simulink model "i2c_logger"  (R2021b)
settings: Solver=FixedStepAuto  StartTime=0.0  StopTime=10.0  RelTol=1e-3  EnableMultiTasking=on
libraries: mbedblockslib x8, simulink x2, realtime_examples_misc x1
settings Model: ExtModeTrigDuration=10  Creator=Robert Viramontes  LastModifiedBy=Robert Viramontes
settings OptimizationCC: EnhancedBackFolding=on  PassReuseOutputArgsAs=Individual arguments  ZeroExternalMemoryAtStartup=off  ZeroInternalMemoryAtStartup=off  MaxStackSize=64  OptimizeBlockOrder=speed  DifferentSizesBufferReuse=on  OptimizationCustomize=off  EfficientTunableParamExpr=on
settings DebuggingCC: ParameterTunabilityLossMsg=error
settings HardwareCC: ProdBitPerPointer=32  ProdBitPerSizeT=32  ProdBitPerPtrDiffT=32  ProdLargestAtomicInteger=Long  ProdLargestAtomicFloat=Double  ProdWordSize=32  ProdHWDeviceType=ARM Compatible->ARM Cortex
settings SFSimCC: MATLABDynamicMemAlloc=off
settings RTWCC: Description=Embedded Coder  SystemTargetFile=ert.tlc  HardwareBoard=STM32 Nucleo F411RE  TemplateMakefile=ert_default_tmf  Toolchain=GNU Tools for ARM Embedded Processors
settings CodeAppCC: ForceParamTrailComments=on  IgnoreCustomStorageClasses=off  OperatorAnnotations=on  SimulinkDataObjDesc=on  SFDataObjDesc=on  InsertBlockDesc=on
settings ERTTargetCC: ExtModeTransport=3  ExtModeStaticAlloc=on  ExtModeStaticAllocSize=2000  ExtModeMexFile=ext_xcp  ExtModeIntrfLevel=Level2 - Open

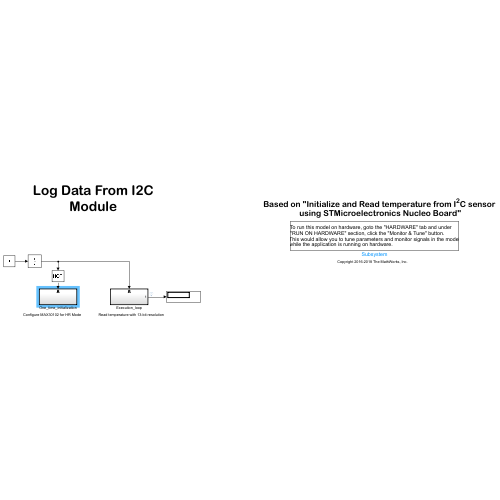
[thumbnail: Simulink's stored preview of the top-level diagram]
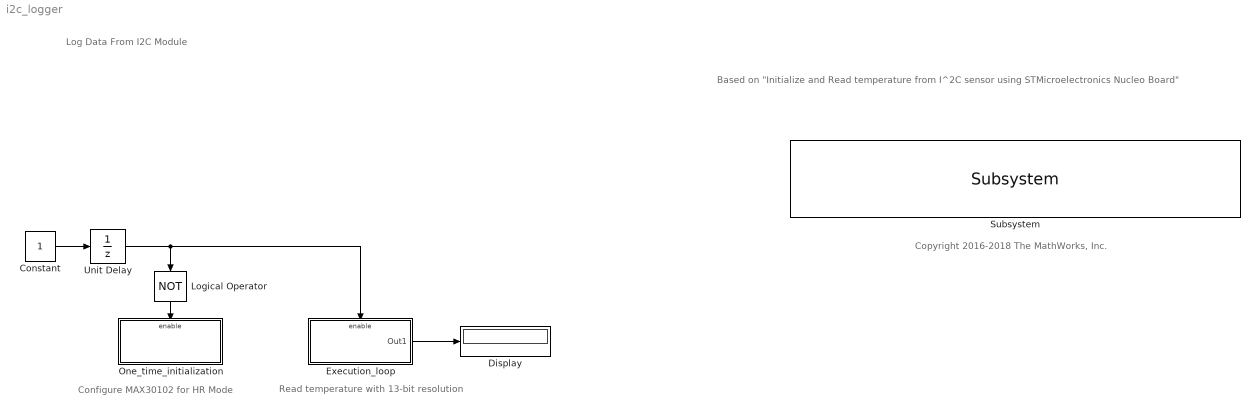
== system i2c_logger ==
  note: Log Data From I2C Module
  note: Read temperature with 13-bit resolution
  note: Configure MAX30102 for HR Mode
  note: Copyright 2016-2018 The MathWorks, Inc.
  note: Based on "Initialize and Read temperature from I^2C sensor
      |  using STMicroelectronics Nucleo Board"
  Constant : Constant  OutDataTypeStr=boolean  SampleTime=0.1
  Display : Display
      settings: Format=hex (Stored Integer)
  Execution_loop : Subsystem  TreatAsAtomicUnit=on
  Logical Operator : Logic  Operator=NOT  AllPortsSameDT=off  OutDataTypeStr=boolean
  One_time_initialization : Subsystem  TreatAsAtomicUnit=on
  Subsystem : realtime_examples_misc/Subsystem  SystemSampleTime=-1  VariantActivationTime=update diagram  Latency=0  AutoFrameSizeCalculation=off
      settings: SourceProductBaseCode=SL
  Unit Delay : UnitDelay  SampleTime=-1  HasFrameUpgradeWarning=on
  wires:
  Logical Operator/1 -> One_time_initialization/Enable
  Execution_loop/1(Out1) -> Display/1
  Constant/1 -> Unit Delay/1
  Unit Delay/1 -> Execution_loop/Enable, Logical Operator/1

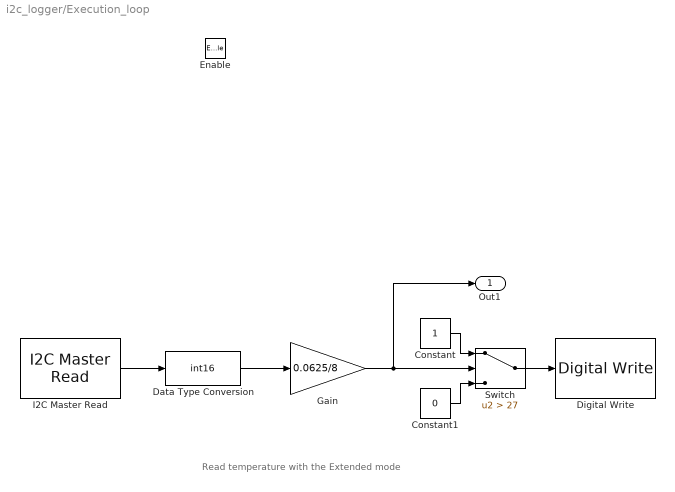
== system i2c_logger/Execution_loop ==
  note: Read temperature with the Extended mode
  Enable : EnablePort
  Constant : Constant  OutDataTypeStr=uint8
  Constant1 : Constant  Value=0  OutDataTypeStr=uint8
  Data Type Conversion : DataTypeConversion  OutDataTypeStr=int16  ConvertRealWorld=Stored Integer (SI)
  Digital Write : mbedblockslib/Digital Write  Pin=13  Direction=output
      settings: SourceProductBaseCode=MICROBIT,NUCLEO,STMICRODIS
  Gain : Gain  Gain=0.0625/8  OutDataTypeStr=single
  I2C Master Read : mbedblockslib/I2C Master Read  I2CModule=0  Mode=Master  SlaveAddress=hex2dec('48')  SlaveByteOrder=BigEndian  Direction=Receiver  RegisterAddressMode=on  RegisterAddress=uint8(0)  SlaveDataType=uint16  DataLength=1  NoAck=off  RepeatedStart=off  OutputStatus=off  SampleTime=0.1
      settings: SourceProductBaseCode=MICROBIT,NUCLEO,STMICRODIS
  Switch : Switch  Criteria=u2 > Threshold  Threshold=27
  Out1 : Outport  InitialOutput=0  VectorParamsAs1DForOutWhenUnconnected=off
  wires:
  I2C Master Read/1 -> Data Type Conversion/1
  Data Type Conversion/1 -> Gain/1
  Gain/1 -> Out1/1, Switch/2
  Constant/1 -> Switch/1
  Constant1/1 -> Switch/3
  Switch/1 -> Digital Write/1

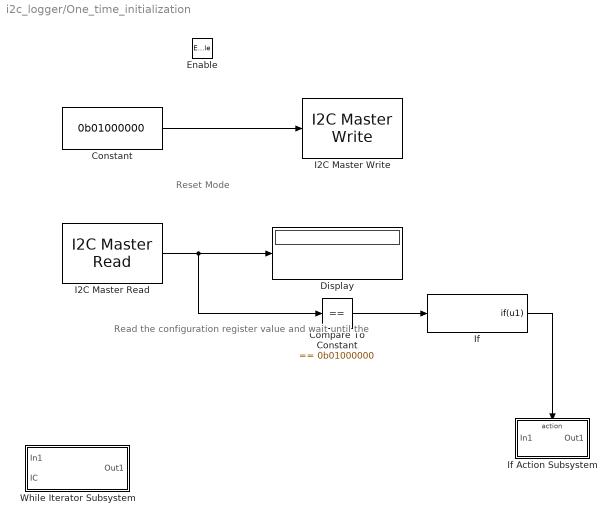
== system i2c_logger/One_time_initialization ==
  note: Reset Mode
  note: Read the configuration register value and wait until the
  Enable : EnablePort
  Compare To Constant : simulink/Logic and Bit Operations/Compare To Constant  relop===  const=0b01000000  OutDataTypeStr=boolean
  Constant : Constant  Value=0b01000000  OutDataTypeStr=uint8
  Display : Display
  I2C Master Read : mbedblockslib/I2C Master Read  I2CModule=0  Mode=Master  SlaveAddress=hex2dec('57')  SlaveByteOrder=BigEndian  Direction=Receiver  RegisterAddressMode=on  RegisterAddress=uint8(0x09)  SlaveDataType=uint8  DataLength=1  NoAck=off  RepeatedStart=off  OutputStatus=off  SampleTime=0.1
      settings: SourceProductBaseCode=MICROBIT,NUCLEO,STMICRODIS
  I2C Master Write : mbedblockslib/I2C Master Write  I2CModule=0  Mode=Master  SlaveAddress=0x57  SlaveByteOrder=BigEndian  Direction=Transmitter  RegisterAddressMode=on  RegisterAddress=uint8(0x09)  SlaveDataType=uint8  DataLength=2  NoAck=off  RepeatedStart=off  OutputStatus=off
      settings: SourceProductBaseCode=MICROBIT,NUCLEO,STMICRODIS
  If : If  IfExpression=u1  ShowElse=off
  If Action Subsystem : Subsystem  TreatAsAtomicUnit=on
  While Iterator Subsystem : Subsystem  TreatAsAtomicUnit=on
  wires:
  Constant/1 -> I2C Master Write/1
  I2C Master Read/1 -> Compare To Constant/1, Display/1
  Compare To Constant/1 -> If/1
  If/1 -> If Action Subsystem/Action

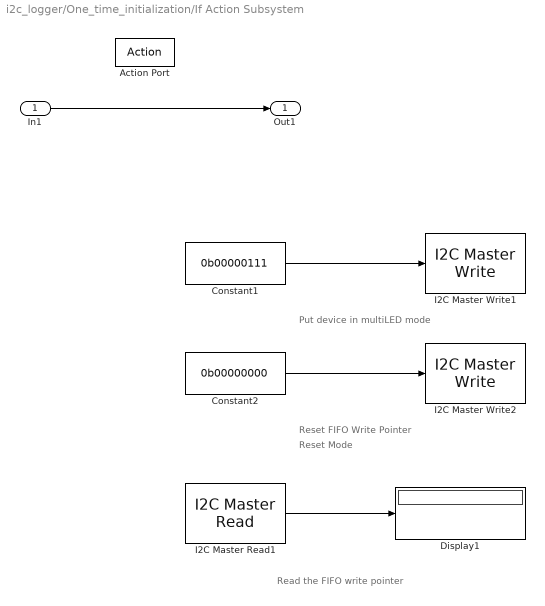
== system i2c_logger/One_time_initialization/If Action Subsystem ==
  note: Read the FIFO write pointer
  note: Reset Mode
  note: Put device in multiLED mode
  note: Reset FIFO Write Pointer
  In1 : Inport
  Action Port : ActionPort  ActionPortLabel=if(u1)
  Constant1 : Constant  Value=0b00000111  OutDataTypeStr=uint8
  Constant2 : Constant  Value=0b00000000  OutDataTypeStr=uint8
  Display1 : Display
  I2C Master Read1 : mbedblockslib/I2C Master Read  I2CModule=0  Mode=Master  SlaveAddress=hex2dec('57')  SlaveByteOrder=BigEndian  Direction=Receiver  RegisterAddressMode=on  RegisterAddress=uint8(0x04)  SlaveDataType=uint8  DataLength=1  NoAck=off  RepeatedStart=off  OutputStatus=off  SampleTime=0.1
      settings: SourceProductBaseCode=MICROBIT,NUCLEO,STMICRODIS
  I2C Master Write1 : mbedblockslib/I2C Master Write  I2CModule=0  Mode=Master  SlaveAddress=0x57  SlaveByteOrder=BigEndian  Direction=Transmitter  RegisterAddressMode=on  RegisterAddress=uint8(0x09)  SlaveDataType=uint8  DataLength=2  NoAck=off  RepeatedStart=off  OutputStatus=off
      settings: SourceProductBaseCode=MICROBIT,NUCLEO,STMICRODIS
  I2C Master Write2 : mbedblockslib/I2C Master Write  I2CModule=0  Mode=Master  SlaveAddress=0x57  SlaveByteOrder=BigEndian  Direction=Transmitter  RegisterAddressMode=on  RegisterAddress=uint8(0x04)  SlaveDataType=uint8  DataLength=2  NoAck=off  RepeatedStart=off  OutputStatus=off
      settings: SourceProductBaseCode=MICROBIT,NUCLEO,STMICRODIS
  Out1 : Outport
  wires:
  In1/1 -> Out1/1
  I2C Master Read1/1 -> Display1/1
  Constant2/1 -> I2C Master Write2/1
  Constant1/1 -> I2C Master Write1/1

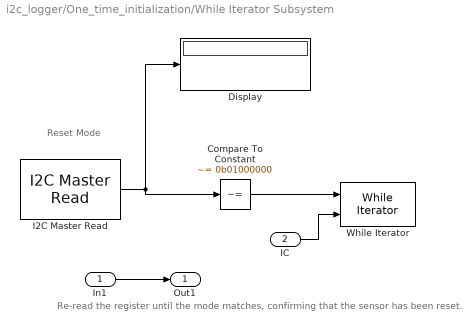
== system i2c_logger/One_time_initialization/While Iterator Subsystem ==
  note: Reset Mode
  note: Re-read the register until the mode matches, confirming that the sensor has been reset.
  In1 : Inport
  IC : Inport  Port=2
  Compare To Constant : simulink/Logic and Bit Operations/Compare To Constant  relop=~=  const=0b01000000  OutDataTypeStr=boolean
  Display : Display
  I2C Master Read : mbedblockslib/I2C Master Read  I2CModule=0  Mode=Master  SlaveAddress=hex2dec('57')  SlaveByteOrder=BigEndian  Direction=Receiver  RegisterAddressMode=on  RegisterAddress=uint8(0x09)  SlaveDataType=uint8  DataLength=1  NoAck=off  RepeatedStart=off  OutputStatus=off  SampleTime=0.1
      settings: SourceProductBaseCode=MICROBIT,NUCLEO,STMICRODIS
  While Iterator : WhileIterator  MaxIters=10
  Out1 : Outport
  wires:
  I2C Master Read/1 -> Display/1, Compare To Constant/1
  Compare To Constant/1 -> While Iterator/1
  IC/1 -> While Iterator/2
  In1/1 -> Out1/1
